simulink model "verify"  (R2017a)
settings: Solver=VariableStepAuto  StartTime=0.0  StopTime=10.0  RelTol=1e-3
values from neighbouring files (symbols this model uses):
  dm = 2.96e-5    (= 2.96e-05)    [dataEx1.m]
  J = 2.37e-5    (= 2.37e-05)    [dataEx1.m]
  Ke = 1 / sc * 60 / 2 / pi    (= 0.0697028947848)    [dataEx1.m]
  Ki = c*c*(Ke*Kt+R*dm+P*Kt)^2 / Kt/J/R    (= 123.951819086)    [dataEx1.m]
  Kp = (2*c-1)*(Ke*Kt+R*dm)/Kt + 2*c*P    (= 4.22806805686)    [dataEx1.m]
  Kt = 69.7e-3    (= 0.0697)    [dataEx1.m]
  L = 11.4e-3    (= 0.0114)    [dataEx1.m]
  R = 112    [dataEx1.m]    (also in discreteVelocity.m = poly2sym([1,-1],z))
  t0 = J*R*(Kt*Ke+R*dm+Kt*Ki)/(Kt*c*(Ke*Kt+R*dm+P*Kt))    (= 2.17472288753)    [dataEx1.m]
  Tc = 1e-3    (= 0.001)    [dataEx1.m]
undefined symbols (not defined in the file or in its folder): P_design
libraries: simulink x2, cstblocks x1
settings Model: Creator=99641  LastModifiedBy=99641

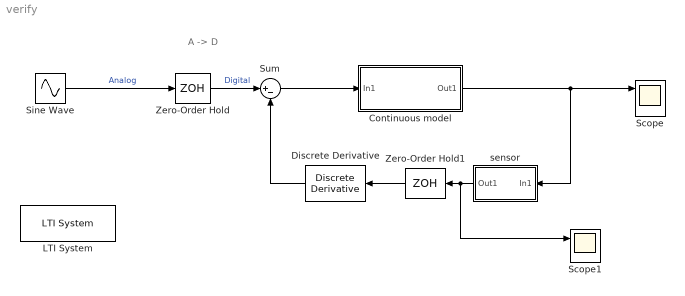
== system verify ==
  note: A -> D
  Continuous model : Subsystem
  Discrete Derivative : simulink/Discrete/Discrete Derivative  gainval=1.0  ICPrevScaledInput=0.0  OutMin=[]  OutMax=[]  OutDataType=fixdt(1, 16)  OutScaling=2^-10  DoSatur=off
  LTI System : cstblocks/LTI System  sys=tf(1,[1 1])  IC=[]
  Scope : Scope  NumInputPorts=2
  Scope1 : Scope  NumInputPorts=2
  Sine Wave : Sin  Amplitude=20  SampleTime=0
  Sum : Sum  Inputs=|+-
  Zero-Order Hold : ZeroOrderHold  SampleTime=0.002
  Zero-Order Hold1 : ZeroOrderHold  SampleTime=-1
  sensor : Subsystem
  wires:
  Sine Wave/1 -> Zero-Order Hold/1  "Analog"
  Zero-Order Hold/1 -> Sum/1  "Digital"
  Sum/1 -> Continuous model/1(In1)
  Continuous model/1(Out1) -> sensor/1(In1), Scope/1
  sensor/1(Out1) -> Scope1/1, Zero-Order Hold1/1
  Zero-Order Hold1/1 -> Discrete Derivative/1
  Discrete Derivative/1 -> Sum/2

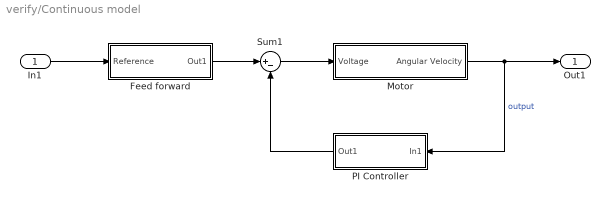
== system verify/Continuous model ==
  In1 : Inport
  "Feed forward " : Subsystem
  "Motor     " : Subsystem
  "PI Controller " : Subsystem
  Sum1 : Sum  Inputs=|+-
  Out1 : Outport
  wires:
  "Motor     "/1(Angular Velocity) -> Out1/1, "PI Controller "/1(In1)  "output"
  Sum1/1 -> "Motor     "/1(Voltage)
  "PI Controller "/1(Out1) -> Sum1/2
  "Feed forward "/1(Out1) -> Sum1/1
  In1/1 -> "Feed forward "/1(Reference)

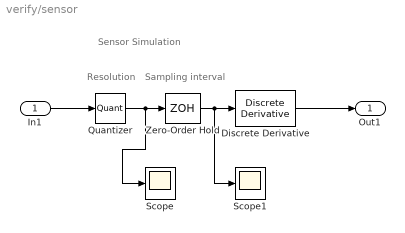
== system verify/sensor ==
  note: Sensor Simulation
  note: Resolution
  note: Sampling interval
  In1 : Inport
  Discrete Derivative : simulink/Discrete/Discrete Derivative  gainval=1.0  ICPrevScaledInput=0.0  InputProcessing=Inherited  OutMin=[]  OutMax=[]  OutDataType=fixdt(1, 16)  OutScaling=2^-10  DoSatur=off
  Quantizer : Quantizer  QuantizationInterval=2*pi/8192
  Scope : Scope
  Scope1 : Scope
  Zero-Order Hold : ZeroOrderHold  SampleTime=0.01
  Out1 : Outport
  wires:
  Zero-Order Hold/1 -> Scope1/1, Discrete Derivative/1
  Quantizer/1 -> Scope/1, Zero-Order Hold/1
  Discrete Derivative/1 -> Out1/1
  In1/1 -> Quantizer/1

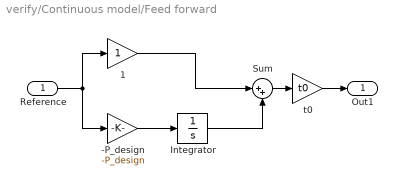
== system verify/Continuous model/Feed forward  ==
  Reference : Inport
  "-P_design " : Gain  Gain=-P_design
  "1 " : Gain
  Integrator : Integrator
  Sum : Sum  Inputs=|++
  t0 : Gain  Gain=t0
  Out1 : Outport
  wires:
  Reference/1 -> "-P_design "/1, "1 "/1
  "1 "/1 -> Sum/1
  Integrator/1 -> Sum/2
  "-P_design "/1 -> Integrator/1
  Sum/1 -> t0/1
  t0/1 -> Out1/1

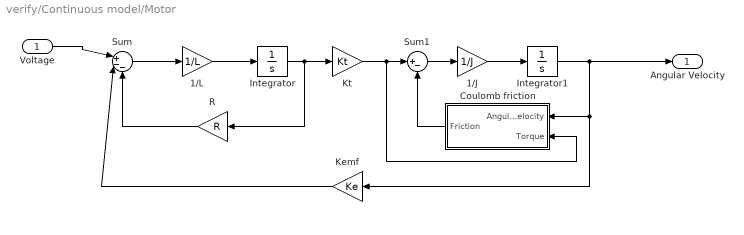
== system verify/Continuous model/Motor      ==
  Voltage : Inport
  1/J : Gain  Gain=1/J
  1/L : Gain  Gain=1/L
  Coulomb friction : Subsystem
  Integrator : Integrator
  Integrator1 : Integrator
  Kemf : Gain  Gain=Ke
  "Kt " : Gain  Gain=Kt
  R : Gain  Gain=R
  Sum : Sum  Inputs=|+--
  Sum1 : Sum  Inputs=|+-
  Angular Velocity : Outport
  wires:
  Sum/1 -> 1/L/1
  Voltage/1 -> Sum/1
  R/1 -> Sum/3
  1/J/1 -> Integrator1/1
  "Kt "/1 -> Coulomb friction/2("Torque "), Sum1/1
  Sum1/1 -> 1/J/1
  Integrator1/1 -> Angular Velocity/1, Kemf/1, Coulomb friction/1(Angular Velocity)
  1/L/1 -> Integrator/1
  Integrator/1 -> R/1, "Kt "/1
  Kemf/1 -> Sum/2
  Coulomb friction/1("Friction ") -> Sum1/2

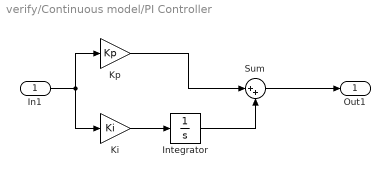
== system verify/Continuous model/PI Controller  ==
  In1 : Inport
  Integrator : Integrator
  "Ki " : Gain  Gain=Ki
  Kp : Gain  Gain=Kp
  Sum : Sum  Inputs=|++
  Out1 : Outport
  wires:
  Sum/1 -> Out1/1
  "Ki "/1 -> Integrator/1
  Integrator/1 -> Sum/2
  Kp/1 -> Sum/1
  In1/1 -> Kp/1, "Ki "/1

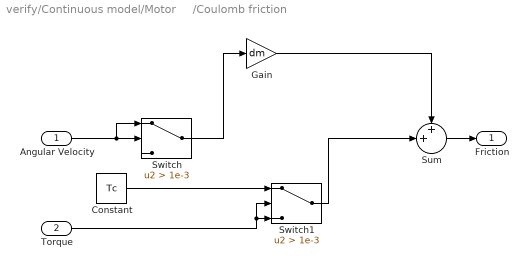
== system verify/Continuous model/Motor     /Coulomb friction ==
  Angular Velocity : Inport
  "Torque " : Inport  Port=2
  Constant : Constant  Value=Tc
  Gain : Gain  Gain=dm
  Sum : Sum  Inputs=++|
  Switch : Switch  Criteria=u2 > Threshold  Threshold=1e-3
  Switch1 : Switch  Criteria=u2 > Threshold  Threshold=1e-3
  "Friction " : Outport
  wires:
  Switch1/1 -> Sum/2
  Gain/1 -> Sum/1
  Sum/1 -> "Friction "/1
  Angular Velocity/1 -> Switch/1, Switch/2
  Switch/1 -> Gain/1
  "Torque "/1 -> Switch1/3, Switch1/2
  Constant/1 -> Switch1/1
